simulink library "courseFollow_cl"  (R2018b)
settings: Solver=VariableStepAuto  StartTime=0.0  StopTime=10.0  RelTol=1e-3
values from neighbouring files (symbols this model uses):
  V = [-sin(phi1).*cos(lambda1), -sin(lambda1) ... (first row only)    [plotFigure8.m]
libraries: dspmathops x4, dspinverses x3, vectorNormalizer_ul x2
settings Model: Creator=James Reed  LastModifiedBy=James Reed

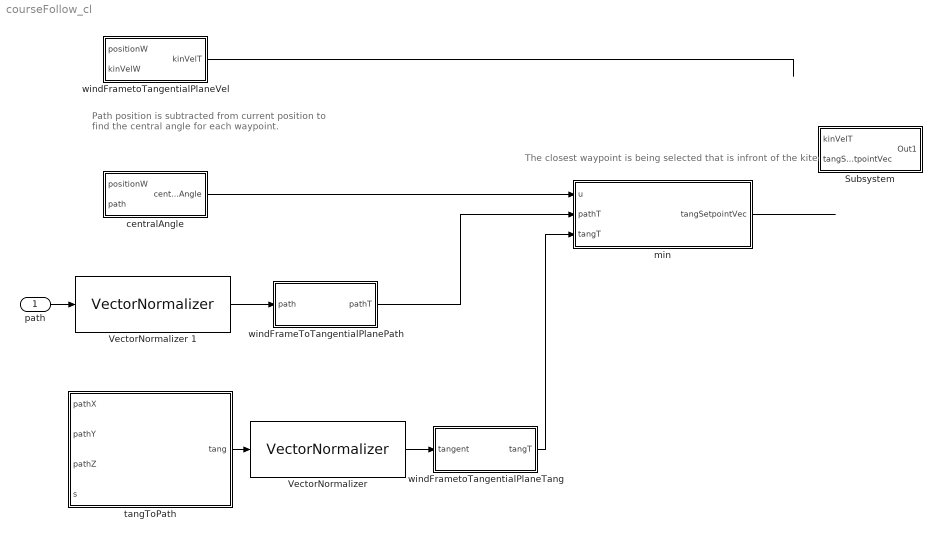
== system courseFollow_cl ==
  note: The closest waypoint is being selected that is infront of
      | the kite
  note: Path position is subtracted from current
      | position to find the central angle for each
      | waypoint.
  path : Inport
  Subsystem : Subsystem
  "VectorNormalizer " : vectorNormalizer_ul/VectorNormalizer   SystemSampleTime=-1
  VectorNormalizer 1 : vectorNormalizer_ul/VectorNormalizer   SystemSampleTime=-1
  centralAngle : Subsystem
  min : MATLAB Function  TreatAsAtomicUnit=on
  tangToPath : Subsystem
  windFrameToTangentialPlanePath : Subsystem
  windFrametoTangentialPlaneTang : Subsystem
  windFrametoTangentialPlaneVel : Subsystem
  wires:
  tangToPath/1(tang) -> "VectorNormalizer "/1
  "VectorNormalizer "/1 -> windFrametoTangentialPlaneTang/1("tangent ")
  centralAngle/1("centralAngle ") -> min/1(u)
  min/1(tangSetpointVec) -> ?
  windFrametoTangentialPlaneTang/1(tangT) -> min/3(tangT)
  path/1 -> VectorNormalizer 1/1
  VectorNormalizer 1/1 -> windFrameToTangentialPlanePath/1("path ")
  windFrameToTangentialPlanePath/1(pathT) -> min/2(pathT)
  windFrametoTangentialPlaneVel/1(kinVelT) -> ?

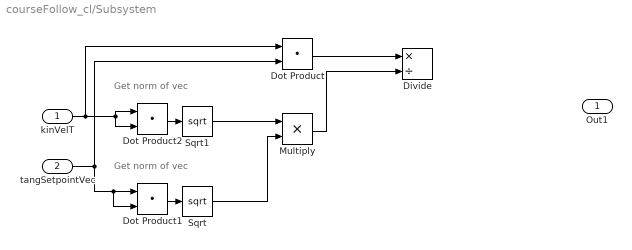
== system courseFollow_cl/Subsystem ==
  note: Get norm of vec
  note: Get norm of vec
  kinVelT : Inport
  tangSetpointVec : Inport  Port=2
  Divide : Product  Inputs=*/
  Dot Product : DotProduct  InputSameDT=on  OutDataTypeStr=Inherit: Inherit via internal rule
  Dot Product1 : DotProduct  InputSameDT=on  OutDataTypeStr=Inherit: Inherit via internal rule
  Dot Product2 : DotProduct  InputSameDT=on  OutDataTypeStr=Inherit: Inherit via internal rule
  Multiply : Product
  Sqrt : Sqrt  SaturateOnIntegerOverflow=on
  Sqrt1 : Sqrt  SaturateOnIntegerOverflow=on
  Out1 : Outport
  wires:
  Sqrt/1 -> Multiply/2
  Dot Product1/1 -> Sqrt/1
  tangSetpointVec/1 -> Dot Product/2, Dot Product1/2, Dot Product1/1
  Sqrt1/1 -> Multiply/1
  Dot Product2/1 -> Sqrt1/1
  kinVelT/1 -> Dot Product/1, Dot Product2/2, Dot Product2/1
  Dot Product/1 -> Divide/1
  Multiply/1 -> Divide/2

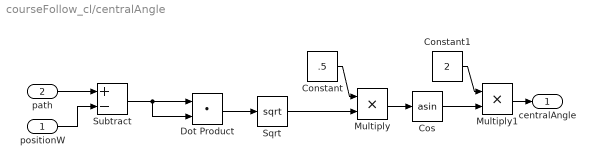
== system courseFollow_cl/centralAngle ==
  "positionW " : Inport
  "path " : Inport  Port=2
  Constant : Constant  Value=.5
  Constant1 : Constant  Value=2
  Cos : Trigonometry  Operator=asin
  Dot Product : DotProduct  InputSameDT=on  OutDataTypeStr=Inherit: Inherit via internal rule
  Multiply : Product
  Multiply1 : Product
  Sqrt : Sqrt  SaturateOnIntegerOverflow=on
  Subtract : Sum  Inputs=+-
  "centralAngle " : Outport
  wires:
  Constant/1 -> Multiply/1
  Multiply/1 -> Cos/1
  "path "/1 -> Subtract/1
  Cos/1 -> Multiply1/2
  Constant1/1 -> Multiply1/1
  Multiply1/1 -> "centralAngle "/1
  "positionW "/1 -> Subtract/2
  Sqrt/1 -> Multiply/2
  Subtract/1 -> Dot Product/2, Dot Product/1
  Dot Product/1 -> Sqrt/1

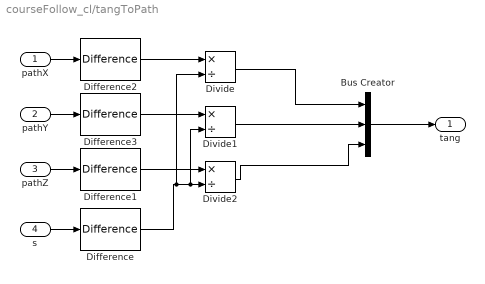
== system courseFollow_cl/tangToPath ==
  "pathX " : Inport
  pathY : Inport  Port=2
  pathZ : Inport  Port=3
  "s " : Inport  Port=4
  Bus Creator : BusCreator  Inputs=3
  Difference{,1..3} (4 alike) : dspmathops/Difference  Run=No  dim=Columns  Dimension=1  roundingMode=Floor  overflowMode=off  outputDataTypeStr=Inherit: Same as accumulator  outputMin=[]  outputMax=[]  outputLastDataTypeStr=Inherit: Same as accumulator
      settings: SourceProductName=DSP System Toolbox  SourceProductBaseCode=DS
  Divide : Product  Inputs=*/
  Divide1 : Product  Inputs=*/
  Divide2 : Product  Inputs=*/
  tang : Outport
  wires:
  Divide1/1 -> Bus Creator/2
  Divide/1 -> Bus Creator/1
  Bus Creator/1 -> tang/1
  Divide2/1 -> Bus Creator/3
  "pathX "/1 -> Difference2/1
  Difference1/1 -> Divide2/1
  Difference2/1 -> Divide/1
  Difference/1 -> Divide/2, Divide1/2, Divide2/2
  pathZ/1 -> Difference1/1
  Difference3/1 -> Divide1/1
  pathY/1 -> Difference3/1
  "s "/1 -> Difference/1

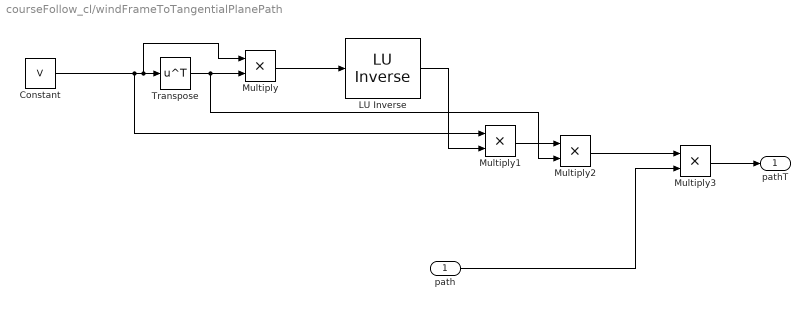
== system courseFollow_cl/windFrameToTangentialPlanePath ==
  "path " : Inport
  " LU Inverse" : dspinverses/ LU Inverse
      settings: SourceProductName=DSP System Toolbox
  Constant : Constant  Value=V
  Multiply{,1..3} (4 alike) : Product
  Transpose : Math  Operator=transpose  SaturateOnIntegerOverflow=on
  pathT : Outport
  wires:
  Multiply1/1 -> Multiply2/1
  Multiply2/1 -> Multiply3/1
  Constant/1 -> Multiply1/1, Multiply/1, Transpose/1
  " LU Inverse"/1 -> Multiply1/2
  Multiply3/1 -> pathT/1
  "path "/1 -> Multiply3/2
  Transpose/1 -> Multiply2/2, Multiply/2
  Multiply/1 -> " LU Inverse"/1

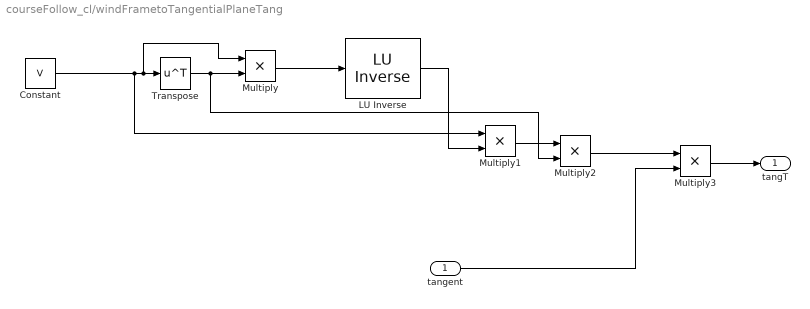
== system courseFollow_cl/windFrametoTangentialPlaneTang ==
  "tangent " : Inport
  " LU Inverse" : dspinverses/ LU Inverse
      settings: SourceProductName=DSP System Toolbox
  Constant : Constant  Value=V
  Multiply{,1..3} (4 alike) : Product
  Transpose : Math  Operator=transpose  SaturateOnIntegerOverflow=on
  tangT : Outport
  wires:
  Multiply/1 -> " LU Inverse"/1
  Transpose/1 -> Multiply2/2, Multiply/2
  Multiply3/1 -> tangT/1
  Multiply2/1 -> Multiply3/1
  " LU Inverse"/1 -> Multiply1/2
  Constant/1 -> Multiply1/1, Multiply/1, Transpose/1
  Multiply1/1 -> Multiply2/1
  "tangent "/1 -> Multiply3/2

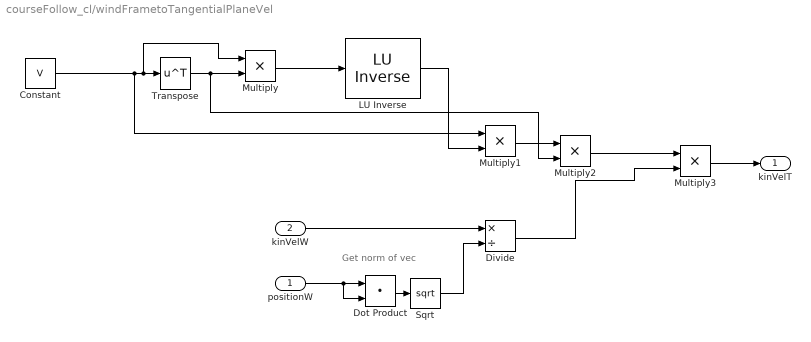
== system courseFollow_cl/windFrametoTangentialPlaneVel ==
  note: Get norm of vec
  positionW : Inport
  kinVelW : Inport  Port=2
  " LU Inverse" : dspinverses/ LU Inverse
      settings: SourceProductName=DSP System Toolbox
  Constant : Constant  Value=V
  Divide : Product  Inputs=*/
  Dot Product : DotProduct  InputSameDT=on  OutDataTypeStr=Inherit: Inherit via internal rule
  Multiply{,1..3} (4 alike) : Product
  Sqrt : Sqrt  SaturateOnIntegerOverflow=on
  Transpose : Math  Operator=transpose  SaturateOnIntegerOverflow=on
  kinVelT : Outport
  wires:
  " LU Inverse"/1 -> Multiply1/2
  Multiply1/1 -> Multiply2/1
  Multiply/1 -> " LU Inverse"/1
  Constant/1 -> Multiply1/1, Multiply/1, Transpose/1
  Multiply3/1 -> kinVelT/1
  Multiply2/1 -> Multiply3/1
  Divide/1 -> Multiply3/2
  Transpose/1 -> Multiply2/2, Multiply/2
  positionW/1 -> Dot Product/2, Dot Product/1
  kinVelW/1 -> Divide/1
  Sqrt/1 -> Divide/2
  Dot Product/1 -> Sqrt/1

== matlab function courseFollow_cl/min ==
  data: u input; pathT input; tangSetpointVec output; tangT input
function tangSetpointVec = fcn(u,pathT,tangT)

[val,idx] = min(u);



tangSetpointVec = tangT(idx);
